simulink model "IP_Core_SS_Switch_and_PWM"  (R2021a)
settings: Solver=VariableStepAuto  StartTime=0.0  StopTime=0.001  RelTol=1e-3
values from neighbouring files (symbols this model uses):
  f_FPGA_clk = 100e6    (= 100000000)    [Init_IP_Core.m]
  T_FPGA_clk = 1/f_FPGA_clk    (= 1e-08)    [Init_IP_Core.m]
libraries: hdlsllib x4, simulink x2
(part 1 of 3)
settings Model: Creator=BHK  LastModifiedBy=micha
settings SolverCC: AlgebraicLoopSolver=TrustRegion
settings DataIOCC: ReturnWorkspaceOutputs=off
settings OptimizationCC: BlockReduction=off  ConditionallyExecuteInputs=off  DefaultParameterBehavior=Inlined
settings DebuggingCC: AlgebraicLoopMsg=error  SFMachineParentedDataDiag=warning  ArithmeticOperatorsInVariantConditions=warning
settings HardwareCC: ProdBitPerPointer=32  ProdBitPerSizeT=32  ProdBitPerPtrDiffT=32  ProdLargestAtomicFloat=None  ProdIntDivRoundTo=Undefined  ProdEndianess=Unspecified  ProdWordSize=32  ProdHWDeviceType=ASIC/FPGA->ASIC/FPGA  TargetBitPerPointer=64  TargetBitPerSizeT=64  TargetBitPerPtrDiffT=64  TargetLongLongMode=on  TargetIntDivRoundTo=Zero  TargetEndianess=LittleEndian  TargetWordSize=64  TargetHWDeviceType=Custom Processor->MATLAB Host Computer  ProdEqTarget=off
settings SFSimCC: SimUseLocalCustomCode=off  CustomCodeUndefinedFunction=UseInterfaceOnly
settings RTWCC: RTWUseLocalCustomCode=off

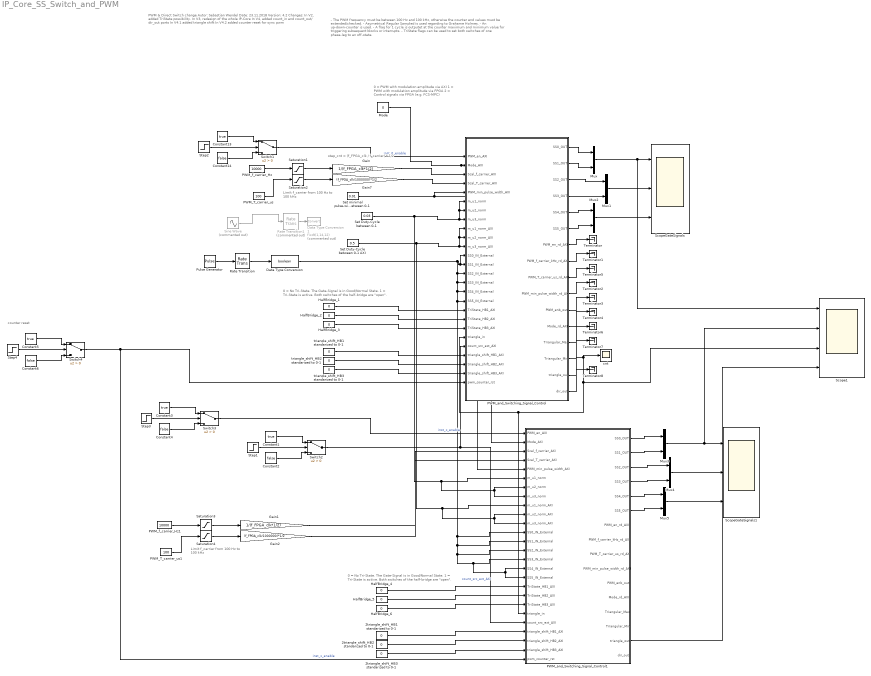
== system IP_Core_SS_Switch_and_PWM ==
  note: counter reset
  note: 0 = No Tri-State. The Gate-Signal is in Good/Normal State.
      | 1 = Tri-State is active. Both switches of the half-bridge are "open".
  note: PWM & Direct Switch change
      |
      | Autor: Sebastian Wendel
      | Date: 23.11.2018
      | Version: 4.2
      | Changes: In V2, added TriState possibility.
      | In V3, redesign of the whole IP-Core
      | In V4, added count_in and count_out/
      | dir_out ports
      | In V4.1 added triangle shift
      | In V4.2 added counter reset for sync pwm
  note: 0 = PWM with modulation amplitude via AXI
      | 1 = PWM with modulation amplitude via FPGA
      | 2 = Control signals via FPGA (e.g. FCS-MPC)
  note: step_cnt = (f_FPGA_clk / f_carrier) * 1/2
  note: Limit f_carrier from
      | 100 Hz to 100 kHz
  note: - The PWM frequency must be between 100 Hz and 100 kHz, otherwise the counter end values must be extended/checked.
      | - Asymetrical Regular Sampled is used regarding to Grahame Holmes.
      | - An up-down-counter is used.
      | - A flag for 1 cycle is outputet at the counter maximum and minimum value for triggering subsequent blocks or interrupts.
      | - TriState flags can be used to set both switches of one phase-leg to an off-state.
  note: 0 = No Tri-State. The Gate-Signal is in Good/Normal State.
      | 1 = Tri-State is active. Both switches of the half-bridge are "open".
  note: Limit f_carrier from
      | 100 Hz to 100 kHz
  2triangle_shift_HB1 standarized to 0-1 : Constant  Value=0  OutDataTypeStr=fixdt(0,18,17)  SampleTime=T_FPGA_clk
  2triangle_shift_HB2 standarized to 0-1 : Constant  Value=0  OutDataTypeStr=fixdt(0,18,17)  SampleTime=T_FPGA_clk
  2triangle_shift_HB3 standarized to 0-1 : Constant  Value=0  OutDataTypeStr=fixdt(0,18,17)  SampleTime=T_FPGA_clk
  Constant{1,3,5,13} (4 alike) : Constant  Value=true  SampleTime=T_FPGA_clk
  Constant{2,4,6,14} (4 alike) : Constant  Value=false  SampleTime=T_FPGA_clk
  Data Type Conversion : DataTypeConversion  OutDataTypeStr=boolean
  Data Type Conversion1 : DataTypeConversion  Commented=on  OutDataTypeStr=fixdt(1,14,12)
  Gain : Gain  Gain=1/(f_FPGA_clk*1/2)  OutDataTypeStr=fixdt(0,25,26)
  Gain1 : Gain  Gain=1/(f_FPGA_clk*1/2)  OutDataTypeStr=fixdt(0,25,26)
  Gain2 : Gain  Gain=(f_FPGA_clk/1000000)*1/2  OutDataTypeStr=fixdt(0,25,0)
  Gain7 : Gain  Gain=(f_FPGA_clk/1000000)*1/2  OutDataTypeStr=fixdt(0,25,0)
  HalfBridge_{1..6} (6 alike) : Constant  Value=0  OutDataTypeStr=fixdt(0,2,0)  SampleTime=T_FPGA_clk
  Mode : Constant  Value=0  OutDataTypeStr=fixdt(0,2,0)  SampleTime=T_FPGA_clk
  Mux{,1..5} (6 alike) : Mux  Inputs=2
  PWM_T_carrier_us : Constant  Value=100  OutDataTypeStr=uint32  SampleTime=T_FPGA_clk
  PWM_T_carrier_us1 : Constant  Value=100  OutDataTypeStr=uint32  SampleTime=T_FPGA_clk
  PWM_and_Switching_Signal_Control : Subsystem  TreatAsAtomicUnit=on
  PWM_and_Switching_Signal_Control1 : Subsystem  TreatAsAtomicUnit=on
  PWM_f_carrier_Hz : Constant  Value=10000  OutDataTypeStr=uint32  SampleTime=T_FPGA_clk
  PWM_f_carrier_Hz1 : Constant  Value=10000  OutDataTypeStr=uint32  SampleTime=T_FPGA_clk
  Pulse Generator : DiscretePulseGenerator  PulseType=Time based  Period=0.01  PulseWidth=5
  Rate Transition : RateTransition  OutPortSampleTime=T_FPGA_clk
  Rate Transition1 : RateTransition  Commented=on  OutPortSampleTime=T_FPGA_clk
  Saturation1 : Saturate  UpperLimit=100000  LowerLimit=100
  Saturation2 : Saturate  UpperLimit=10000  LowerLimit=10
  Saturation3 : Saturate  UpperLimit=100000  LowerLimit=100
  Saturation4 : Saturate  UpperLimit=10000  LowerLimit=10
  Scope1 : Scope  NumInputPorts=4
  ScopeGateSignals : Scope  NumInputPorts=3
  ScopeGateSignals1 : Scope  NumInputPorts=3
  Set Duty-Cycle between 0-1 : Constant  Value=0.03  OutDataTypeStr=fixdt(1,14,12)  SampleTime=T_FPGA_clk
  Set Duty-Cycle between 0-1 AXI : Constant  Value=0.5  OutDataTypeStr=fixdt(1,14,12)  SampleTime=T_FPGA_clk
  Set minimal pulse-width between 0-1 : Constant  Value=0.01  OutDataTypeStr=fixdt(1,18,16)  SampleTime=T_FPGA_clk
  Sine Wave : Sin  Commented=on  Frequency=500  SampleTime=0
  Step1 : Step  Time=0.002  After=0  SampleTime=T_FPGA_clk
  Step2 : Step  Time=0.00010  SampleTime=T_FPGA_clk
  Step3 : Step  Time=0.00019  SampleTime=T_FPGA_clk
  Step4 : Step  Time=0.0004  SampleTime=T_FPGA_clk
  Switch{1..4} (4 alike) : Switch  Criteria=u2 > Threshold
  Terminator{,1..8} (9 alike) : Terminator
  cnt : Scope
  triangle_shift_HB1 standarized to 0-1 : Constant  Value=0  OutDataTypeStr=fixdt(0,18,17)  SampleTime=T_FPGA_clk
  triangle_shift_HB2 standarized to 0-1 : Constant  Value=0  OutDataTypeStr=fixdt(0,18,17)  SampleTime=T_FPGA_clk
  triangle_shift_HB3 standarized to 0-1 : Constant  Value=0  OutDataTypeStr=fixdt(0,18,17)  SampleTime=T_FPGA_clk
  wires:
  Step2/1 -> Switch1/2
  Constant13/1 -> Switch1/1
  Constant14/1 -> Switch1/3
  Switch1/1 -> PWM_and_Switching_Signal_Control/1(PWM_en_AXI)  "inst_0_enable"
  Mode/1 -> PWM_and_Switching_Signal_Control1/2(Mode_AXI), PWM_and_Switching_Signal_Control/2(Mode_AXI)
  PWM_f_carrier_Hz/1 -> Saturation1/1
  Set minimal pulse-width between 0-1/1 -> PWM_and_Switching_Signal_Control1/5(PWM_min_pulse_width_AXI), PWM_and_Switching_Signal_Control/5(PWM_min_pulse_width_AXI)
  Sine Wave/1 -> Rate Transition1/1
  PWM_and_Switching_Signal_Control/7(PWM_en_rd_AXI) -> Terminator/1
  PWM_and_Switching_Signal_Control/8(PWM_f_carrier_kHz_rd_AXI) -> Terminator1/1
  PWM_and_Switching_Signal_Control/10(PWM_min_pulse_width_rd_AXI) -> Terminator2/1
  PWM_and_Switching_Signal_Control/11(PWM_enb_out) -> Terminator3/1
  PWM_and_Switching_Signal_Control/12(Mode_rd_AXI) -> Terminator4/1
  Set Duty-Cycle between 0-1 AXI/1 -> PWM_and_Switching_Signal_Control1/11(m_u3_norm_AXI), PWM_and_Switching_Signal_Control1/10(m_u2_norm_AXI), PWM_and_Switching_Signal_Control1/9(m_u1_norm_AXI), PWM_and_Switching_Signal_Control/9(m_u1_norm_AXI), PWM_and_Switching_Signal_Control/10(m_u2_norm_AXI), PWM_and_Switching_Signal_Control/11(m_u3_norm_AXI)
  PWM_and_Switching_Signal_Control/1(SS0_OUT) -> Mux/1
  PWM_and_Switching_Signal_Control/2(SS1_OUT) -> Mux/2
  Mux/1 -> Scope1/1, ScopeGateSignals/1
  PWM_and_Switching_Signal_Control/3(SS2_OUT) -> Mux1/1
  PWM_and_Switching_Signal_Control/4(SS3_OUT) -> Mux1/2
  PWM_and_Switching_Signal_Control/5(SS4_OUT) -> Mux2/1
  PWM_and_Switching_Signal_Control/6(SS5_OUT) -> Mux2/2
  Mux2/1 -> ScopeGateSignals/3
  Mux1/1 -> ScopeGateSignals/2
  PWM_T_carrier_us/1 -> Saturation2/1
  Rate Transition/1 -> Data Type Conversion/1
  Pulse Generator/1 -> Rate Transition/1
  PWM_and_Switching_Signal_Control/9(PWM_T_carrier_us_rd_AXI) -> Terminator5/1
  PWM_and_Switching_Signal_Control/13(Triangular_Max) -> Terminator6/1
  HalfBridge_3/1 -> PWM_and_Switching_Signal_Control/20(TriState_HB3_AXI)
  HalfBridge_2/1 -> PWM_and_Switching_Signal_Control/19(TriState_HB2_AXI)
  HalfBridge_1/1 -> PWM_and_Switching_Signal_Control/18(TriState_HB1_AXI)
  PWM_and_Switching_Signal_Control/14(Triangular_Min) -> Terminator7/1
  Gain/1 -> PWM_and_Switching_Signal_Control/3(Scal_f_carrier_AXI)
  Gain7/1 -> PWM_and_Switching_Signal_Control/4(Scal_T_carrier_AXI)
  Saturation1/1 -> Gain/1
  Saturation2/1 -> Gain7/1
  Rate Transition1/1 -> Data Type Conversion1/1
  Set Duty-Cycle between 0-1/1 -> PWM_and_Switching_Signal_Control/6(m_u1_norm), PWM_and_Switching_Signal_Control/7(m_u2_norm), PWM_and_Switching_Signal_Control/8(m_u3_norm), PWM_and_Switching_Signal_Control1/6(m_u1_norm), PWM_and_Switching_Signal_Control1/8(m_u3_norm), PWM_and_Switching_Signal_Control1/7(m_u2_norm)
  PWM_and_Switching_Signal_Control/16(dir_out) -> Terminator8/1
  Constant2/1 -> Switch2/3
  Step1/1 -> Switch2/2
  Constant1/1 -> Switch2/1
  Switch2/1 -> PWM_and_Switching_Signal_Control1/22(count_src_ext_AXI), PWM_and_Switching_Signal_Control/22(count_src_ext_AXI)  "count_src_ext_AXI"
  PWM_and_Switching_Signal_Control/15(triangle_out) -> cnt/1, PWM_and_Switching_Signal_Control/21(triangle_in), PWM_and_Switching_Signal_Control1/21(triangle_in), Scope1/3
  Data Type Conversion/1 -> PWM_and_Switching_Signal_Control/12(SS0_IN_External), PWM_and_Switching_Signal_Control/13(SS1_IN_External), PWM_and_Switching_Signal_Control1/12(SS0_IN_External), PWM_and_Switching_Signal_Control1/13(SS1_IN_External), PWM_and_Switching_Signal_Control1/14(SS2_IN_External), PWM_and_Switching_Signal_Control1/17(SS5_IN_External), PWM_and_Switching_Signal_Control1/16(SS4_IN_External), PWM_and_Switching_Signal_Control1/15(SS3_IN_External), PWM_and_Switching_Signal_Control/17(SS5_IN_External), PWM_and_Switching_Signal_Control/16(SS4_IN_External), PWM_and_Switching_Signal_Control/15(SS3_IN_External), PWM_and_Switching_Signal_Control/14(SS2_IN_External)
  HalfBridge_4/1 -> PWM_and_Switching_Signal_Control1/18(TriState_HB1_AXI)
  HalfBridge_6/1 -> PWM_and_Switching_Signal_Control1/20(TriState_HB3_AXI)
  HalfBridge_5/1 -> PWM_and_Switching_Signal_Control1/19(TriState_HB2_AXI)
  Mux3/1 -> ScopeGateSignals1/1, Scope1/2
  Mux5/1 -> ScopeGateSignals1/3
  Mux4/1 -> ScopeGateSignals1/2
  triangle_shift_HB1 standarized to 0-1/1 -> PWM_and_Switching_Signal_Control/23(triangle_shift_HB1_AXI)
  triangle_shift_HB2 standarized to 0-1/1 -> PWM_and_Switching_Signal_Control/24(triangle_shift_HB2_AXI)
  triangle_shift_HB3 standarized to 0-1/1 -> PWM_and_Switching_Signal_Control/25(triangle_shift_HB3_AXI)
  2triangle_shift_HB1 standarized to 0-1/1 -> PWM_and_Switching_Signal_Control1/23(triangle_shift_HB1_AXI)
  2triangle_shift_HB2 standarized to 0-1/1 -> PWM_and_Switching_Signal_Control1/24(triangle_shift_HB2_AXI)
  2triangle_shift_HB3 standarized to 0-1/1 -> PWM_and_Switching_Signal_Control1/25(triangle_shift_HB3_AXI)
  PWM_and_Switching_Signal_Control1/1(SS0_OUT) -> Mux3/1
  PWM_and_Switching_Signal_Control1/2(SS1_OUT) -> Mux3/2
  PWM_and_Switching_Signal_Control1/3(SS2_OUT) -> Mux4/1
  PWM_and_Switching_Signal_Control1/4(SS3_OUT) -> Mux4/2
  PWM_and_Switching_Signal_Control1/5(SS4_OUT) -> Mux5/1
  PWM_and_Switching_Signal_Control1/6(SS5_OUT) -> Mux5/2
  Step3/1 -> Switch3/2
  Constant4/1 -> Switch3/3
  Constant3/1 -> Switch3/1
  Switch3/1 -> PWM_and_Switching_Signal_Control1/1(PWM_en_AXI)  "inst_x_enable"
  Saturation3/1 -> Gain1/1
  PWM_f_carrier_Hz1/1 -> Saturation3/1
  Saturation4/1 -> Gain2/1
  PWM_T_carrier_us1/1 -> Saturation4/1
  Gain1/1 -> PWM_and_Switching_Signal_Control1/3(Scal_f_carrier_AXI)
  Gain2/1 -> PWM_and_Switching_Signal_Control1/4(Scal_T_carrier_AXI)
  PWM_and_Switching_Signal_Control1/15(triangle_out) -> Scope1/4
  Step4/1 -> Switch4/2
  Constant6/1 -> Switch4/3
  Constant5/1 -> Switch4/1
  Switch4/1 -> PWM_and_Switching_Signal_Control1/26(pwm_counter_rst), PWM_and_Switching_Signal_Control/26(pwm_counter_rst)  "inst_x_enable"

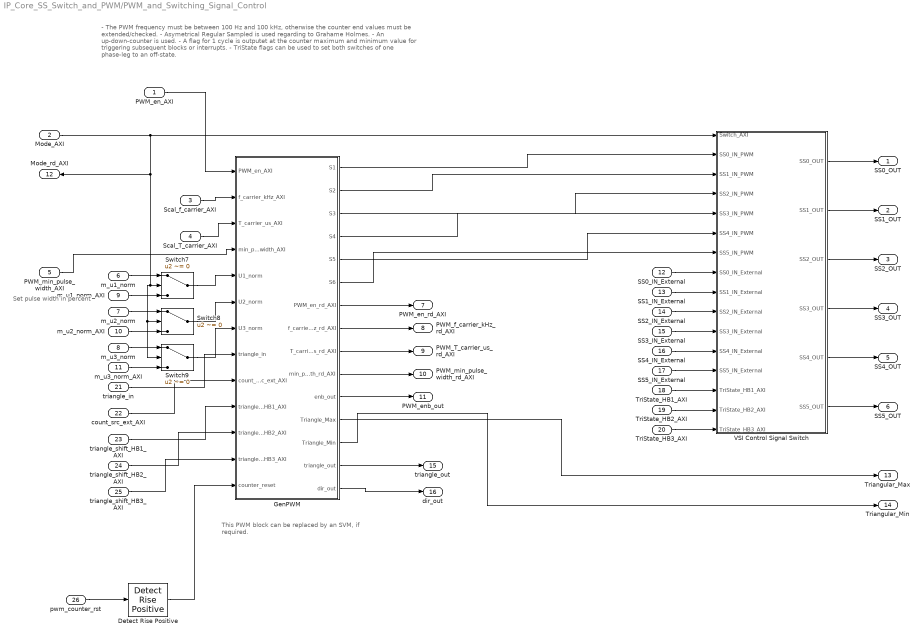
== system IP_Core_SS_Switch_and_PWM/PWM_and_Switching_Signal_Control ==
  note: This PWM block can be replaced by an SVM,
      | if required.
  note: - The PWM frequency must be between 100 Hz and 100 kHz, otherwise the counter end values must be extended/checked.
      | - Asymetrical Regular Sampled is used regarding to Grahame Holmes.
      | - An up-down-counter is used.
      | - A flag for 1 cycle is outputet at the counter maximum and minimum value for triggering subsequent blocks or interrupts.
      | - TriState flags can be used to set both switches of one phase-leg to an off-state.
  note: Set pulse width in percent
  PWM_en_AXI : Inport
  Mode_AXI : Inport  Port=2
  Scal_f_carrier_AXI : Inport  Port=3
  Scal_T_carrier_AXI : Inport  Port=4
  PWM_min_pulse_width_AXI : Inport  Port=5
  m_u1_norm : Inport  Port=6
  m_u2_norm : Inport  Port=7
  m_u3_norm : Inport  Port=8
  m_u1_norm_AXI : Inport  Port=9
  m_u2_norm_AXI : Inport  Port=10
  m_u3_norm_AXI : Inport  Port=11
  SS0_IN_External : Inport  Port=12
  SS1_IN_External : Inport  Port=13
  SS2_IN_External : Inport  Port=14
  SS3_IN_External : Inport  Port=15
  SS4_IN_External : Inport  Port=16
  SS5_IN_External : Inport  Port=17
  TriState_HB1_AXI : Inport  Port=18
  TriState_HB2_AXI : Inport  Port=19
  TriState_HB3_AXI : Inport  Port=20
  triangle_in : Inport  Port=21
  count_src_ext_AXI : Inport  Port=22
  triangle_shift_HB1_AXI : Inport  Port=23
  triangle_shift_HB2_AXI : Inport  Port=24
  triangle_shift_HB3_AXI : Inport  Port=25
  pwm_counter_rst : Inport  Port=26
  Detect Rise Positive : simulink/Logic and Bit Operations/Detect Rise Positive  vinit=0  OutDataTypeStr=boolean
  GenPWM : Subsystem  TreatAsAtomicUnit=on
  Switch7 : Switch  Criteria=u2 ~= 0
  Switch8 : Switch  Criteria=u2 ~= 0
  Switch9 : Switch  Criteria=u2 ~= 0
  VSI Control Signal Switch : Subsystem
  SS0_OUT : Outport  VectorParamsAs1DForOutWhenUnconnected=off
  SS1_OUT : Outport  Port=2  VectorParamsAs1DForOutWhenUnconnected=off
  SS2_OUT : Outport  Port=3  VectorParamsAs1DForOutWhenUnconnected=off
  SS3_OUT : Outport  Port=4  VectorParamsAs1DForOutWhenUnconnected=off
  SS4_OUT : Outport  Port=5  VectorParamsAs1DForOutWhenUnconnected=off
  SS5_OUT : Outport  Port=6  VectorParamsAs1DForOutWhenUnconnected=off
  PWM_en_rd_AXI : Outport  Port=7  VectorParamsAs1DForOutWhenUnconnected=off
  PWM_f_carrier_kHz_rd_AXI : Outport  Port=8  VectorParamsAs1DForOutWhenUnconnected=off
  PWM_T_carrier_us_rd_AXI : Outport  Port=9  VectorParamsAs1DForOutWhenUnconnected=off
  PWM_min_pulse_width_rd_AXI : Outport  Port=10  VectorParamsAs1DForOutWhenUnconnected=off
  PWM_enb_out : Outport  Port=11  VectorParamsAs1DForOutWhenUnconnected=off
  Mode_rd_AXI : Outport  Port=12  VectorParamsAs1DForOutWhenUnconnected=off
  Triangular_Max : Outport  Port=13  VectorParamsAs1DForOutWhenUnconnected=off
  Triangular_Min : Outport  Port=14  VectorParamsAs1DForOutWhenUnconnected=off
  triangle_out : Outport  Port=15  VectorParamsAs1DForOutWhenUnconnected=off
  dir_out : Outport  Port=16  VectorParamsAs1DForOutWhenUnconnected=off
  wires:
  VSI Control Signal Switch/1(SS0_OUT) -> SS0_OUT/1
  Mode_AXI/1 -> Mode_rd_AXI/1, Switch9/2, Switch8/2, Switch7/2, VSI Control Signal Switch/1(Switch_AXI)
  GenPWM/4(S4) -> VSI Control Signal Switch/5(SS3_IN_PWM)
  Scal_f_carrier_AXI/1 -> GenPWM/2(f_carrier_kHz_AXI)
  GenPWM/2(S2) -> VSI Control Signal Switch/3(SS1_IN_PWM)
  SS1_IN_External/1 -> VSI Control Signal Switch/9(SS1_IN_External)
  GenPWM/3(S3) -> VSI Control Signal Switch/4(SS2_IN_PWM)
  GenPWM/5(S5) -> VSI Control Signal Switch/6(SS4_IN_PWM)
  GenPWM/6(S6) -> VSI Control Signal Switch/7(SS5_IN_PWM)
  VSI Control Signal Switch/6(SS5_OUT) -> SS5_OUT/1
  GenPWM/1(S1) -> VSI Control Signal Switch/2(SS0_IN_PWM)
  GenPWM/11(enb_out) -> PWM_enb_out/1
  VSI Control Signal Switch/3(SS2_OUT) -> SS2_OUT/1
  SS3_IN_External/1 -> VSI Control Signal Switch/11(SS3_IN_External)
  SS0_IN_External/1 -> VSI Control Signal Switch/8(SS0_IN_External)
  VSI Control Signal Switch/2(SS1_OUT) -> SS1_OUT/1
  SS4_IN_External/1 -> VSI Control Signal Switch/12(SS4_IN_External)
  SS5_IN_External/1 -> VSI Control Signal Switch/13(SS5_IN_External)
  VSI Control Signal Switch/5(SS4_OUT) -> SS4_OUT/1
  PWM_min_pulse_width_AXI/1 -> GenPWM/4(min_pulse_width_AXI)
  SS2_IN_External/1 -> VSI Control Signal Switch/10(SS2_IN_External)
  VSI Control Signal Switch/4(SS3_OUT) -> SS3_OUT/1
  Switch9/1 -> GenPWM/7(U3_norm)
  m_u1_norm_AXI/1 -> Switch7/3
  m_u1_norm/1 -> Switch7/1
  m_u2_norm/1 -> Switch8/1
  m_u2_norm_AXI/1 -> Switch8/3
  m_u3_norm/1 -> Switch9/1
  m_u3_norm_AXI/1 -> Switch9/3
  GenPWM/7(PWM_en_rd_AXI) -> PWM_en_rd_AXI/1
  GenPWM/8(f_carrier_kHz_rd_AXI) -> PWM_f_carrier_kHz_rd_AXI/1
  GenPWM/10(min_pulse_width_rd_AXI) -> PWM_min_pulse_width_rd_AXI/1
  GenPWM/9(T_carrier_us_rd_AXI) -> PWM_T_carrier_us_rd_AXI/1
  Switch8/1 -> GenPWM/6(U2_norm)
  Switch7/1 -> GenPWM/5(U1_norm)
  Scal_T_carrier_AXI/1 -> GenPWM/3(T_carrier_us_AXI)
  GenPWM/12(Triangle_Max) -> Triangular_Max/1
  TriState_HB1_AXI/1 -> VSI Control Signal Switch/14(TriState_HB1_AXI)
  TriState_HB2_AXI/1 -> VSI Control Signal Switch/15(TriState_HB2_AXI)
  TriState_HB3_AXI/1 -> VSI Control Signal Switch/16(TriState_HB3_AXI)
  GenPWM/13(Triangle_Min) -> Triangular_Min/1
  triangle_in/1 -> GenPWM/8(triangle_in)
  GenPWM/14(triangle_out) -> triangle_out/1
  GenPWM/15(dir_out) -> dir_out/1
  count_src_ext_AXI/1 -> GenPWM/9(count_src_ext_AXI)
  triangle_shift_HB1_AXI/1 -> GenPWM/10(triangle_shift_HB1_AXI)
  triangle_shift_HB3_AXI/1 -> GenPWM/12(triangle_shift_HB3_AXI)
  triangle_shift_HB2_AXI/1 -> GenPWM/11(triangle_shift_HB2_AXI)
  PWM_en_AXI/1 -> GenPWM/1(PWM_en_AXI)
  pwm_counter_rst/1 -> Detect Rise Positive/1
  Detect Rise Positive/1 -> GenPWM/13(counter_reset)

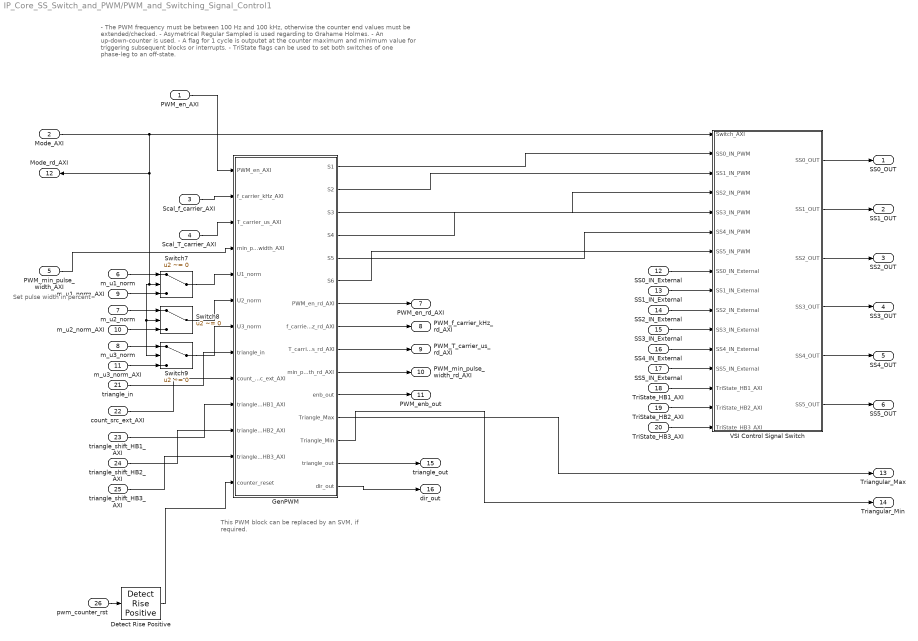
== system IP_Core_SS_Switch_and_PWM/PWM_and_Switching_Signal_Control1 ==
  note: This PWM block can be replaced by an SVM,
      | if required.
  note: - The PWM frequency must be between 100 Hz and 100 kHz, otherwise the counter end values must be extended/checked.
      | - Asymetrical Regular Sampled is used regarding to Grahame Holmes.
      | - An up-down-counter is used.
      | - A flag for 1 cycle is outputet at the counter maximum and minimum value for triggering subsequent blocks or interrupts.
      | - TriState flags can be used to set both switches of one phase-leg to an off-state.
  note: Set pulse width in percent
  PWM_en_AXI : Inport
  Mode_AXI : Inport  Port=2
  Scal_f_carrier_AXI : Inport  Port=3
  Scal_T_carrier_AXI : Inport  Port=4
  PWM_min_pulse_width_AXI : Inport  Port=5
  m_u1_norm : Inport  Port=6
  m_u2_norm : Inport  Port=7
  m_u3_norm : Inport  Port=8
  m_u1_norm_AXI : Inport  Port=9
  m_u2_norm_AXI : Inport  Port=10
  m_u3_norm_AXI : Inport  Port=11
  SS0_IN_External : Inport  Port=12
  SS1_IN_External : Inport  Port=13
  SS2_IN_External : Inport  Port=14
  SS3_IN_External : Inport  Port=15
  SS4_IN_External : Inport  Port=16
  SS5_IN_External : Inport  Port=17
  TriState_HB1_AXI : Inport  Port=18
  TriState_HB2_AXI : Inport  Port=19
  TriState_HB3_AXI : Inport  Port=20
  triangle_in : Inport  Port=21
  count_src_ext_AXI : Inport  Port=22
  triangle_shift_HB1_AXI : Inport  Port=23
  triangle_shift_HB2_AXI : Inport  Port=24
  triangle_shift_HB3_AXI : Inport  Port=25
  pwm_counter_rst : Inport  Port=26
  Detect Rise Positive : simulink/Logic and Bit Operations/Detect Rise Positive  vinit=0  OutDataTypeStr=boolean
  GenPWM : Subsystem  TreatAsAtomicUnit=on
  Switch7 : Switch  Criteria=u2 ~= 0
  Switch8 : Switch  Criteria=u2 ~= 0
  Switch9 : Switch  Criteria=u2 ~= 0
  VSI Control Signal Switch : Subsystem
  SS0_OUT : Outport  VectorParamsAs1DForOutWhenUnconnected=off
  SS1_OUT : Outport  Port=2  VectorParamsAs1DForOutWhenUnconnected=off
  SS2_OUT : Outport  Port=3  VectorParamsAs1DForOutWhenUnconnected=off
  SS3_OUT : Outport  Port=4  VectorParamsAs1DForOutWhenUnconnected=off
  SS4_OUT : Outport  Port=5  VectorParamsAs1DForOutWhenUnconnected=off
  SS5_OUT : Outport  Port=6  VectorParamsAs1DForOutWhenUnconnected=off
  PWM_en_rd_AXI : Outport  Port=7  VectorParamsAs1DForOutWhenUnconnected=off
  PWM_f_carrier_kHz_rd_AXI : Outport  Port=8  VectorParamsAs1DForOutWhenUnconnected=off
  PWM_T_carrier_us_rd_AXI : Outport  Port=9  VectorParamsAs1DForOutWhenUnconnected=off
  PWM_min_pulse_width_rd_AXI : Outport  Port=10  VectorParamsAs1DForOutWhenUnconnected=off
  PWM_enb_out : Outport  Port=11  VectorParamsAs1DForOutWhenUnconnected=off
  Mode_rd_AXI : Outport  Port=12  VectorParamsAs1DForOutWhenUnconnected=off
  Triangular_Max : Outport  Port=13  VectorParamsAs1DForOutWhenUnconnected=off
  Triangular_Min : Outport  Port=14  VectorParamsAs1DForOutWhenUnconnected=off
  triangle_out : Outport  Port=15  VectorParamsAs1DForOutWhenUnconnected=off
  dir_out : Outport  Port=16  VectorParamsAs1DForOutWhenUnconnected=off
  wires:
  VSI Control Signal Switch/1(SS0_OUT) -> SS0_OUT/1
  Mode_AXI/1 -> Mode_rd_AXI/1, Switch9/2, Switch8/2, Switch7/2, VSI Control Signal Switch/1(Switch_AXI)
  GenPWM/4(S4) -> VSI Control Signal Switch/5(SS3_IN_PWM)
  Scal_f_carrier_AXI/1 -> GenPWM/2(f_carrier_kHz_AXI)
  GenPWM/2(S2) -> VSI Control Signal Switch/3(SS1_IN_PWM)
  SS1_IN_External/1 -> VSI Control Signal Switch/9(SS1_IN_External)
  GenPWM/3(S3) -> VSI Control Signal Switch/4(SS2_IN_PWM)
  GenPWM/5(S5) -> VSI Control Signal Switch/6(SS4_IN_PWM)
  GenPWM/6(S6) -> VSI Control Signal Switch/7(SS5_IN_PWM)
  VSI Control Signal Switch/6(SS5_OUT) -> SS5_OUT/1
  GenPWM/1(S1) -> VSI Control Signal Switch/2(SS0_IN_PWM)
  GenPWM/11(enb_out) -> PWM_enb_out/1
  VSI Control Signal Switch/3(SS2_OUT) -> SS2_OUT/1
  SS3_IN_External/1 -> VSI Control Signal Switch/11(SS3_IN_External)
  SS0_IN_External/1 -> VSI Control Signal Switch/8(SS0_IN_External)
  VSI Control Signal Switch/2(SS1_OUT) -> SS1_OUT/1
  SS4_IN_External/1 -> VSI Control Signal Switch/12(SS4_IN_External)
  SS5_IN_External/1 -> VSI Control Signal Switch/13(SS5_IN_External)
  VSI Control Signal Switch/5(SS4_OUT) -> SS4_OUT/1
  PWM_min_pulse_width_AXI/1 -> GenPWM/4(min_pulse_width_AXI)
  SS2_IN_External/1 -> VSI Control Signal Switch/10(SS2_IN_External)
  VSI Control Signal Switch/4(SS3_OUT) -> SS3_OUT/1
  Switch9/1 -> GenPWM/7(U3_norm)
  m_u1_norm_AXI/1 -> Switch7/3
  m_u1_norm/1 -> Switch7/1
  m_u2_norm/1 -> Switch8/1
  m_u2_norm_AXI/1 -> Switch8/3
  m_u3_norm/1 -> Switch9/1
  m_u3_norm_AXI/1 -> Switch9/3
  GenPWM/7(PWM_en_rd_AXI) -> PWM_en_rd_AXI/1
  GenPWM/8(f_carrier_kHz_rd_AXI) -> PWM_f_carrier_kHz_rd_AXI/1
  GenPWM/10(min_pulse_width_rd_AXI) -> PWM_min_pulse_width_rd_AXI/1
  GenPWM/9(T_carrier_us_rd_AXI) -> PWM_T_carrier_us_rd_AXI/1
  Switch8/1 -> GenPWM/6(U2_norm)
  Switch7/1 -> GenPWM/5(U1_norm)
  Scal_T_carrier_AXI/1 -> GenPWM/3(T_carrier_us_AXI)
  GenPWM/12(Triangle_Max) -> Triangular_Max/1
  TriState_HB1_AXI/1 -> VSI Control Signal Switch/14(TriState_HB1_AXI)
  TriState_HB2_AXI/1 -> VSI Control Signal Switch/15(TriState_HB2_AXI)
  TriState_HB3_AXI/1 -> VSI Control Signal Switch/16(TriState_HB3_AXI)
  GenPWM/13(Triangle_Min) -> Triangular_Min/1
  triangle_in/1 -> GenPWM/8(triangle_in)
  GenPWM/14(triangle_out) -> triangle_out/1
  GenPWM/15(dir_out) -> dir_out/1
  triangle_shift_HB1_AXI/1 -> GenPWM/10(triangle_shift_HB1_AXI)
  triangle_shift_HB3_AXI/1 -> GenPWM/12(triangle_shift_HB3_AXI)
  triangle_shift_HB2_AXI/1 -> GenPWM/11(triangle_shift_HB2_AXI)
  pwm_counter_rst/1 -> Detect Rise Positive/1
  PWM_en_AXI/1 -> GenPWM/1(PWM_en_AXI)
  count_src_ext_AXI/1 -> GenPWM/9(count_src_ext_AXI)
  Detect Rise Positive/1 -> GenPWM/13(counter_reset)

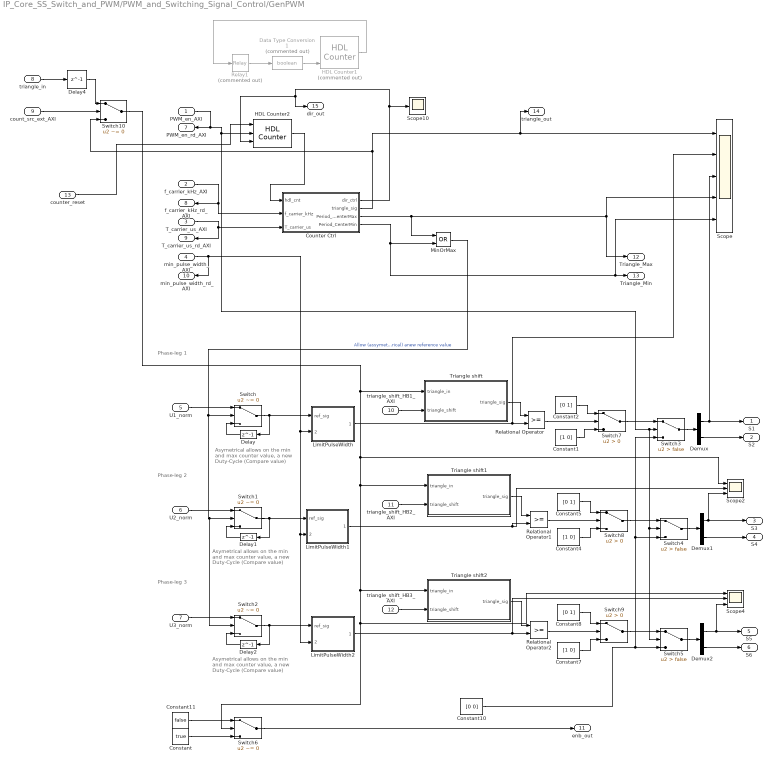
== system IP_Core_SS_Switch_and_PWM/PWM_and_Switching_Signal_Control/GenPWM ==
  note: Asymetrical allows on the min
      |  and max counter value, a new
      |  Duty-Cycle (Compare value)
  note: Phase-leg 1
  note: Phase-leg 2
  note: Phase-leg 3
  note: Asymetrical allows on the min
      |  and max counter value, a new
      |  Duty-Cycle (Compare value)
  note: Asymetrical allows on the min
      |  and max counter value, a new
      |  Duty-Cycle (Compare value)
  PWM_en_AXI : Inport
  f_carrier_kHz_AXI : Inport  Port=2
  T_carrier_us_AXI : Inport  Port=3
  min_pulse_width_AXI : Inport  Port=4
  U1_norm : Inport  Port=5
  U2_norm : Inport  Port=6
  U3_norm : Inport  Port=7
  triangle_in : Inport  Port=8
  count_src_ext_AXI : Inport  Port=9
  triangle_shift_HB1_AXI : Inport  Port=10
  triangle_shift_HB2_AXI : Inport  Port=11
  triangle_shift_HB3_AXI : Inport  Port=12
  counter_reset : Inport  Port=13
  Constant : Constant  Value=true  SampleTime=T_FPGA_clk
  Constant1 : Constant  Value=[1 0]  OutDataTypeStr=fixdt(0,1,0)  SampleTime=T_FPGA_clk
  Constant10 : Constant  Value=[0 0]  OutDataTypeStr=fixdt(0,1,0)  SampleTime=T_FPGA_clk
  Constant11 : Constant  Value=false  SampleTime=T_FPGA_clk
  Constant2 : Constant  Value=[0 1]  OutDataTypeStr=fixdt(0,1,0)  SampleTime=T_FPGA_clk
  Constant4 : Constant  Value=[1 0]  OutDataTypeStr=fixdt(0,1,0)  SampleTime=T_FPGA_clk
  Constant5 : Constant  Value=[0 1]  OutDataTypeStr=fixdt(0,1,0)  SampleTime=T_FPGA_clk
  Constant7 : Constant  Value=[1 0]  OutDataTypeStr=fixdt(0,1,0)  SampleTime=T_FPGA_clk
  Constant8 : Constant  Value=[0 1]  OutDataTypeStr=fixdt(0,1,0)  SampleTime=T_FPGA_clk
  Counter Ctrl : Subsystem
  Data Type Conversion1 : DataTypeConversion  Commented=on  OutDataTypeStr=boolean
  Delay{,1..2,4} (4 alike) : Delay  DelayLength=1
  Demux : Demux  Outputs=2
  Demux1 : Demux  Outputs=2
  Demux2 : Demux  Outputs=2
  HDL Counter1 : hdlsllib/Sources/HDL Counter  Commented=on  CountType=Free running  CountInit=0  CountStep=1  CountMax=100  CountFromType=Initial value  CountFrom=0  CountResetPort=on  CountLoadPort=off  CountEnbPort=on  CountDirPort=on  CountHitOutputPort=off  CountDataType=Signed  CountWordLen=8  CountFracLen=0  CountSampTime=Ts
  HDL Counter2 : hdlsllib/Sources/HDL Counter  CountType=Free running  CountInit=0  CountStep=1  CountMax=100  CountFromType=Initial value  CountFrom=0  CountResetPort=on  CountLoadPort=off  CountEnbPort=on  CountDirPort=on  CountHitOutputPort=off  CountDataType=Unsigned  CountWordLen=20  CountFracLen=0  CountSampTime=1
  LimitPulseWidth : Subsystem
  LimitPulseWidth1 : Subsystem
  LimitPulseWidth2 : Subsystem
  MinOrMax : Logic  Operator=OR  AllPortsSameDT=off  OutDataTypeStr=boolean
  Relational Operator : RelationalOperator  OutDataTypeStr=boolean  RndMeth=Nearest
  Relational Operator1 : RelationalOperator  OutDataTypeStr=boolean  RndMeth=Nearest
  Relational Operator2 : RelationalOperator  OutDataTypeStr=boolean  RndMeth=Nearest
  Relay1 : Relay  Commented=on  OnSwitchValue=100  OffSwitchValue=0  OnOutputValue=0  OffOutputValue=1
  Scope : Scope  NumInputPorts=5
  Scope10 : Scope
  Scope2 : Scope  NumInputPorts=3
  Scope4 : Scope  NumInputPorts=3
  Switch : Switch  Criteria=u2 ~= 0  Threshold=1
  Switch1 : Switch  Criteria=u2 ~= 0
  Switch10 : Switch  Criteria=u2 ~= 0  Threshold=1
  Switch2 : Switch  Criteria=u2 ~= 0
  Switch3 : Switch  Criteria=u2 > Threshold  Threshold=false
  Switch4 : Switch  Criteria=u2 > Threshold  Threshold=false
  Switch5 : Switch  Criteria=u2 > Threshold  Threshold=false
  Switch6 : Switch  Criteria=u2 ~= 0
  Switch7 : Switch  Criteria=u2 > Threshold
  Switch8 : Switch  Criteria=u2 > Threshold
  Switch9 : Switch  Criteria=u2 > Threshold
  Triangle shift : Subsystem
  Triangle shift1 : Subsystem
  Triangle shift2 : Subsystem
  S1 : Outport  VectorParamsAs1DForOutWhenUnconnected=off
  S2 : Outport  Port=2  VectorParamsAs1DForOutWhenUnconnected=off
  S3 : Outport  Port=3  VectorParamsAs1DForOutWhenUnconnected=off
  S4 : Outport  Port=4  VectorParamsAs1DForOutWhenUnconnected=off
  S5 : Outport  Port=5  VectorParamsAs1DForOutWhenUnconnected=off
  S6 : Outport  Port=6  VectorParamsAs1DForOutWhenUnconnected=off
  PWM_en_rd_AXI : Outport  Port=7  VectorParamsAs1DForOutWhenUnconnected=off
  f_carrier_kHz_rd_AXI : Outport  Port=8  VectorParamsAs1DForOutWhenUnconnected=off
  T_carrier_us_rd_AXI : Outport  Port=9  VectorParamsAs1DForOutWhenUnconnected=off
  min_pulse_width_rd_AXI : Outport  Port=10  VectorParamsAs1DForOutWhenUnconnected=off
  enb_out : Outport  Port=11  VectorParamsAs1DForOutWhenUnconnected=off
  Triangle_Max : Outport  Port=12  VectorParamsAs1DForOutWhenUnconnected=off
  Triangle_Min : Outport  Port=13  VectorParamsAs1DForOutWhenUnconnected=off
  triangle_out : Outport  Port=14  VectorParamsAs1DForOutWhenUnconnected=off
  dir_out : Outport  Port=15  VectorParamsAs1DForOutWhenUnconnected=off
  wires:
  Constant7/1 -> Switch9/3
  Demux2/2 -> S6/1
  Constant8/1 -> Switch9/1
  Relational Operator2/1 -> Switch9/2
  Switch9/1 -> Switch5/1
  Demux/2 -> S2/1
  Relational Operator/1 -> Switch7/2
  Demux1/2 -> S4/1
  Constant5/1 -> Switch8/1
  Relational Operator1/1 -> Switch8/2
  Constant4/1 -> Switch8/3
  Constant1/1 -> Switch7/3
  Constant2/1 -> Switch7/1
  LimitPulseWidth/1(ref_sig_limit) -> Scope/2, Relational Operator/2
  LimitPulseWidth1/1(ref_sig_limit) -> Scope2/2, Relational Operator1/2
  LimitPulseWidth2/1(ref_sig_limit) -> Scope4/2, Relational Operator2/2
  Counter Ctrl/2(triangle_sig) -> triangle_out/1, Scope/1, Switch10/3
  PWM_en_AXI/1 -> Switch3/2, Switch4/2, Switch5/2, HDL Counter2/2, PWM_en_rd_AXI/1
  Delay/1 -> Switch/3
  Delay1/1 -> Switch1/3
  Delay2/1 -> Switch2/3
  Switch5/1 -> Demux2/1
  Switch8/1 -> Switch4/1
  Switch4/1 -> Demux1/1
  Switch3/1 -> Demux/1
  Constant10/1 -> Switch5/3, Switch3/3, Switch4/3
  U1_norm/1 -> Switch/1
  U3_norm/1 -> Switch2/1
  U2_norm/1 -> Switch1/1
  Counter Ctrl/1(dir_ctrl) -> dir_out/1, HDL Counter2/3, Scope10/1
  f_carrier_kHz_AXI/1 -> f_carrier_kHz_rd_AXI/1, Counter Ctrl/2(f_carrier_kHz)
  Relay1/1 -> Data Type Conversion1/1
  Data Type Conversion1/1 -> HDL Counter1/3
  HDL Counter1/1 -> Relay1/1
  Switch/1 -> Delay/1, LimitPulseWidth/1(ref_sig)
  Switch1/1 -> LimitPulseWidth1/1(ref_sig), Delay1/1
  Switch2/1 -> LimitPulseWidth2/1(ref_sig), Delay2/1
  Demux/1 -> Scope/3, S1/1
  Switch6/1 -> enb_out/1
  Constant11/1 -> Switch6/1
  Constant/1 -> Switch6/3
  Demux1/1 -> Scope2/3, S3/1
  Demux2/1 -> Scope4/3, S5/1
  T_carrier_us_AXI/1 -> T_carrier_us_rd_AXI/1, Counter Ctrl/3(T_carrier_us)
  Switch7/1 -> Switch3/1
  min_pulse_width_AXI/1 -> LimitPulseWidth/2(min_pulse_width), LimitPulseWidth2/2(min_pulse_width), LimitPulseWidth1/2(min_pulse_width), min_pulse_width_rd_AXI/1
  Counter Ctrl/3(Period_CenterMax) -> MinOrMax/1, Triangle_Max/1, Scope/4
  Counter Ctrl/4(Period_CenterMin) -> MinOrMax/2, Scope/5, Triangle_Min/1
  MinOrMax/1 -> Switch1/2, Switch2/2, Switch/2  "Allow (assymetrical) anew reference value"
  triangle_in/1 -> Delay4/1
  count_src_ext_AXI/1 -> Switch10/2
  HDL Counter2/1 -> Counter Ctrl/1(hdl_cnt)
  Delay4/1 -> Switch10/1
  triangle_shift_HB1_AXI/1 -> Triangle shift/2(triangle_shift)
  Triangle shift/1(triangle_sig) -> Relational Operator/1
  Triangle shift1/1(triangle_sig) -> Relational Operator1/1
  Switch10/1 -> Triangle shift/1(triangle_in), Triangle shift1/1(triangle_in), Triangle shift2/1(triangle_in), Scope4/1, Switch6/2, Scope2/1
  triangle_shift_HB2_AXI/1 -> Triangle shift1/2(triangle_shift)
  Triangle shift2/1(triangle_sig) -> Relational Operator2/1
  triangle_shift_HB3_AXI/1 -> Triangle shift2/2(triangle_shift)
  counter_reset/1 -> HDL Counter2/1

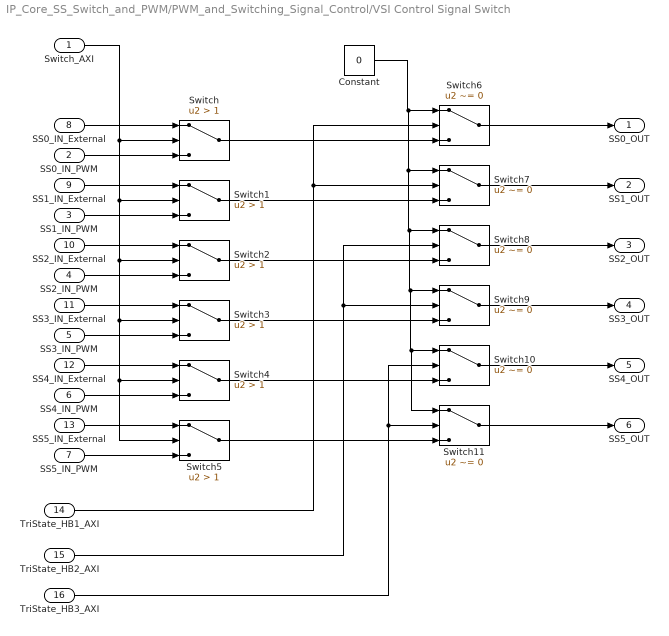
== system IP_Core_SS_Switch_and_PWM/PWM_and_Switching_Signal_Control/VSI Control Signal Switch ==
  Switch_AXI : Inport
  SS0_IN_PWM : Inport  Port=2
  SS1_IN_PWM : Inport  Port=3
  SS2_IN_PWM : Inport  Port=4
  SS3_IN_PWM : Inport  Port=5
  SS4_IN_PWM : Inport  Port=6
  SS5_IN_PWM : Inport  Port=7
  SS0_IN_External : Inport  Port=8
  SS1_IN_External : Inport  Port=9
  SS2_IN_External : Inport  Port=10
  SS3_IN_External : Inport  Port=11
  SS4_IN_External : Inport  Port=12
  SS5_IN_External : Inport  Port=13
  TriState_HB1_AXI : Inport  Port=14
  TriState_HB2_AXI : Inport  Port=15
  TriState_HB3_AXI : Inport  Port=16
  Constant : Constant  Value=0  OutDataTypeStr=boolean  SampleTime=T_FPGA_clk
  Switch{,1..5} (6 alike) : Switch  Criteria=u2 > Threshold  Threshold=1
  Switch{6..11} (6 alike) : Switch  Criteria=u2 ~= 0  Threshold=1
  SS0_OUT : Outport  VectorParamsAs1DForOutWhenUnconnected=off
  SS1_OUT : Outport  Port=2  VectorParamsAs1DForOutWhenUnconnected=off
  SS2_OUT : Outport  Port=3  VectorParamsAs1DForOutWhenUnconnected=off
  SS3_OUT : Outport  Port=4  VectorParamsAs1DForOutWhenUnconnected=off
  SS4_OUT : Outport  Port=5  VectorParamsAs1DForOutWhenUnconnected=off
  SS5_OUT : Outport  Port=6  VectorParamsAs1DForOutWhenUnconnected=off
  wires:
  Switch_AXI/1 -> Switch4/2, Switch5/2, Switch3/2, Switch2/2, Switch1/2, Switch/2
  Switch5/1 -> Switch11/3
  Switch/1 -> Switch6/3
  Switch3/1 -> Switch9/3
  Switch2/1 -> Switch8/3
  Switch1/1 -> Switch7/3
  Switch4/1 -> Switch10/3
  SS0_IN_PWM/1 -> Switch/3
  SS0_IN_External/1 -> Switch/1
  SS1_IN_External/1 -> Switch1/1
  SS1_IN_PWM/1 -> Switch1/3
  SS2_IN_External/1 -> Switch2/1
  SS2_IN_PWM/1 -> Switch2/3
  SS3_IN_External/1 -> Switch3/1
  SS3_IN_PWM/1 -> Switch3/3
  SS4_IN_External/1 -> Switch4/1
  SS4_IN_PWM/1 -> Switch4/3
  SS5_IN_External/1 -> Switch5/1
  SS5_IN_PWM/1 -> Switch5/3
  TriState_HB3_AXI/1 -> Switch10/2, Switch11/2
  TriState_HB2_AXI/1 -> Switch8/2, Switch9/2
  TriState_HB1_AXI/1 -> Switch6/2, Switch7/2
  Switch11/1 -> SS5_OUT/1
  Switch10/1 -> SS4_OUT/1
  Switch9/1 -> SS3_OUT/1
  Switch8/1 -> SS2_OUT/1
  Switch7/1 -> SS1_OUT/1
  Switch6/1 -> SS0_OUT/1
  Constant/1 -> Switch11/1, Switch10/1, Switch9/1, Switch8/1, Switch7/1, Switch6/1

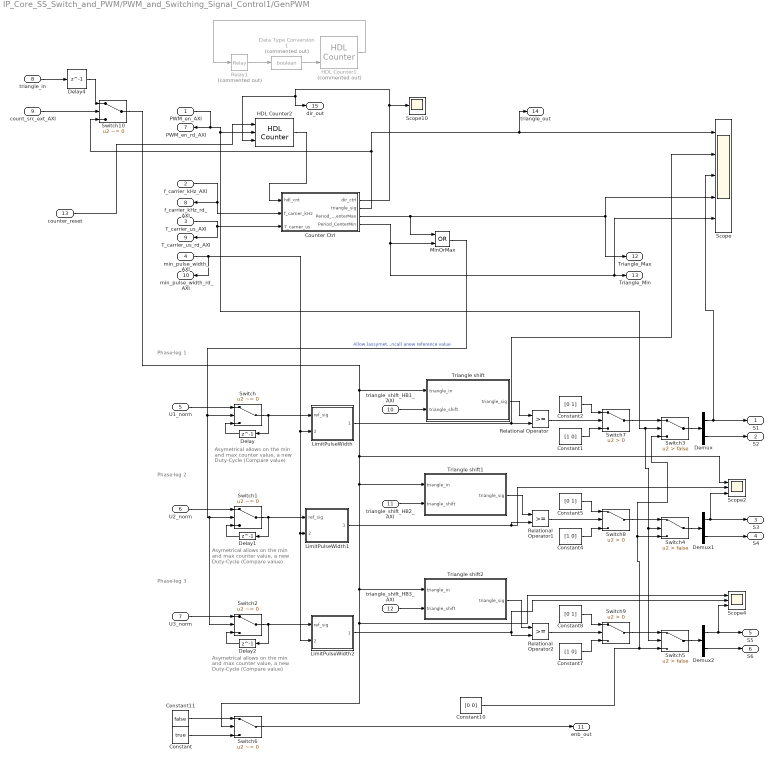
== system IP_Core_SS_Switch_and_PWM/PWM_and_Switching_Signal_Control1/GenPWM ==
  note: Asymetrical allows on the min
      |  and max counter value, a new
      |  Duty-Cycle (Compare value)
  note: Phase-leg 1
  note: Phase-leg 2
  note: Phase-leg 3
  note: Asymetrical allows on the min
      |  and max counter value, a new
      |  Duty-Cycle (Compare value)
  note: Asymetrical allows on the min
      |  and max counter value, a new
      |  Duty-Cycle (Compare value)
  PWM_en_AXI : Inport
  f_carrier_kHz_AXI : Inport  Port=2
  T_carrier_us_AXI : Inport  Port=3
  min_pulse_width_AXI : Inport  Port=4
  U1_norm : Inport  Port=5
  U2_norm : Inport  Port=6
  U3_norm : Inport  Port=7
  triangle_in : Inport  Port=8
  count_src_ext_AXI : Inport  Port=9
  triangle_shift_HB1_AXI : Inport  Port=10
  triangle_shift_HB2_AXI : Inport  Port=11
  triangle_shift_HB3_AXI : Inport  Port=12
  counter_reset : Inport  Port=13
  Constant : Constant  Value=true  SampleTime=T_FPGA_clk
  Constant1 : Constant  Value=[1 0]  OutDataTypeStr=fixdt(0,1,0)  SampleTime=T_FPGA_clk
  Constant10 : Constant  Value=[0 0]  OutDataTypeStr=fixdt(0,1,0)  SampleTime=T_FPGA_clk
  Constant11 : Constant  Value=false  SampleTime=T_FPGA_clk
  Constant2 : Constant  Value=[0 1]  OutDataTypeStr=fixdt(0,1,0)  SampleTime=T_FPGA_clk
  Constant4 : Constant  Value=[1 0]  OutDataTypeStr=fixdt(0,1,0)  SampleTime=T_FPGA_clk
  Constant5 : Constant  Value=[0 1]  OutDataTypeStr=fixdt(0,1,0)  SampleTime=T_FPGA_clk
  Constant7 : Constant  Value=[1 0]  OutDataTypeStr=fixdt(0,1,0)  SampleTime=T_FPGA_clk
  Constant8 : Constant  Value=[0 1]  OutDataTypeStr=fixdt(0,1,0)  SampleTime=T_FPGA_clk
  Counter Ctrl : Subsystem
  Data Type Conversion1 : DataTypeConversion  Commented=on  OutDataTypeStr=boolean
  Delay{,1..2,4} (4 alike) : Delay  DelayLength=1
  Demux : Demux  Outputs=2
  Demux1 : Demux  Outputs=2
  Demux2 : Demux  Outputs=2
  HDL Counter1 : hdlsllib/Sources/HDL Counter  Commented=on  CountType=Free running  CountInit=0  CountStep=1  CountMax=100  CountFromType=Initial value  CountFrom=0  CountResetPort=on  CountLoadPort=off  CountEnbPort=on  CountDirPort=on  CountHitOutputPort=off  CountDataType=Signed  CountWordLen=8  CountFracLen=0  CountSampTime=Ts
  HDL Counter2 : hdlsllib/Sources/HDL Counter  CountType=Free running  CountInit=0  CountStep=1  CountMax=100  CountFromType=Initial value  CountFrom=0  CountResetPort=on  CountLoadPort=off  CountEnbPort=on  CountDirPort=on  CountHitOutputPort=off  CountDataType=Unsigned  CountWordLen=20  CountFracLen=0  CountSampTime=1
  LimitPulseWidth : Subsystem
  LimitPulseWidth1 : Subsystem
  LimitPulseWidth2 : Subsystem
  MinOrMax : Logic  Operator=OR  AllPortsSameDT=off  OutDataTypeStr=boolean
  Relational Operator : RelationalOperator  OutDataTypeStr=boolean  RndMeth=Nearest
  Relational Operator1 : RelationalOperator  OutDataTypeStr=boolean  RndMeth=Nearest
  Relational Operator2 : RelationalOperator  OutDataTypeStr=boolean  RndMeth=Nearest
  Relay1 : Relay  Commented=on  OnSwitchValue=100  OffSwitchValue=0  OnOutputValue=0  OffOutputValue=1
  Scope : Scope  NumInputPorts=5
  Scope10 : Scope
  Scope2 : Scope  NumInputPorts=3
  Scope4 : Scope  NumInputPorts=3
  Switch : Switch  Criteria=u2 ~= 0  Threshold=1
  Switch1 : Switch  Criteria=u2 ~= 0
  Switch10 : Switch  Criteria=u2 ~= 0  Threshold=1
  Switch2 : Switch  Criteria=u2 ~= 0
  Switch3 : Switch  Criteria=u2 > Threshold  Threshold=false
  Switch4 : Switch  Criteria=u2 > Threshold  Threshold=false
  Switch5 : Switch  Criteria=u2 > Threshold  Threshold=false
  Switch6 : Switch  Criteria=u2 ~= 0
  Switch7 : Switch  Criteria=u2 > Threshold
  Switch8 : Switch  Criteria=u2 > Threshold
  Switch9 : Switch  Criteria=u2 > Threshold
  Triangle shift : Subsystem
  Triangle shift1 : Subsystem
  Triangle shift2 : Subsystem
  S1 : Outport  VectorParamsAs1DForOutWhenUnconnected=off
  S2 : Outport  Port=2  VectorParamsAs1DForOutWhenUnconnected=off
  S3 : Outport  Port=3  VectorParamsAs1DForOutWhenUnconnected=off
  S4 : Outport  Port=4  VectorParamsAs1DForOutWhenUnconnected=off
  S5 : Outport  Port=5  VectorParamsAs1DForOutWhenUnconnected=off
  S6 : Outport  Port=6  VectorParamsAs1DForOutWhenUnconnected=off
  PWM_en_rd_AXI : Outport  Port=7  VectorParamsAs1DForOutWhenUnconnected=off
  f_carrier_kHz_rd_AXI : Outport  Port=8  VectorParamsAs1DForOutWhenUnconnected=off
  T_carrier_us_rd_AXI : Outport  Port=9  VectorParamsAs1DForOutWhenUnconnected=off
  min_pulse_width_rd_AXI : Outport  Port=10  VectorParamsAs1DForOutWhenUnconnected=off
  enb_out : Outport  Port=11  VectorParamsAs1DForOutWhenUnconnected=off
  Triangle_Max : Outport  Port=12  VectorParamsAs1DForOutWhenUnconnected=off
  Triangle_Min : Outport  Port=13  VectorParamsAs1DForOutWhenUnconnected=off
  triangle_out : Outport  Port=14  VectorParamsAs1DForOutWhenUnconnected=off
  dir_out : Outport  Port=15  VectorParamsAs1DForOutWhenUnconnected=off
  wires:
  Constant7/1 -> Switch9/3
  Demux2/2 -> S6/1
  Constant8/1 -> Switch9/1
  Relational Operator2/1 -> Switch9/2
  Switch9/1 -> Switch5/1
  Demux/2 -> S2/1
  Relational Operator/1 -> Switch7/2
  Demux1/2 -> S4/1
  Constant5/1 -> Switch8/1
  Relational Operator1/1 -> Switch8/2
  Constant4/1 -> Switch8/3
  Constant1/1 -> Switch7/3
  Constant2/1 -> Switch7/1
  LimitPulseWidth/1(ref_sig_limit) -> Scope/2, Relational Operator/2
  LimitPulseWidth1/1(ref_sig_limit) -> Scope2/2, Relational Operator1/2
  LimitPulseWidth2/1(ref_sig_limit) -> Scope4/2, Relational Operator2/2
  Counter Ctrl/2(triangle_sig) -> triangle_out/1, Scope/1, Switch10/3
  PWM_en_AXI/1 -> Switch3/2, Switch5/2, Switch4/2, HDL Counter2/2, PWM_en_rd_AXI/1
  Delay/1 -> Switch/3
  Delay1/1 -> Switch1/3
  Delay2/1 -> Switch2/3
  Switch5/1 -> Demux2/1
  Switch8/1 -> Switch4/1
  Switch4/1 -> Demux1/1
  Switch3/1 -> Demux/1
  Constant10/1 -> Switch5/3, Switch3/3, Switch4/3
  U1_norm/1 -> Switch/1
  U3_norm/1 -> Switch2/1
  U2_norm/1 -> Switch1/1
  Counter Ctrl/1(dir_ctrl) -> dir_out/1, HDL Counter2/3, Scope10/1
  f_carrier_kHz_AXI/1 -> f_carrier_kHz_rd_AXI/1, Counter Ctrl/2(f_carrier_kHz)
  Relay1/1 -> Data Type Conversion1/1
  Data Type Conversion1/1 -> HDL Counter1/3
  HDL Counter1/1 -> Relay1/1
  Switch/1 -> Delay/1, LimitPulseWidth/1(ref_sig)
  Switch1/1 -> LimitPulseWidth1/1(ref_sig), Delay1/1
  Switch2/1 -> LimitPulseWidth2/1(ref_sig), Delay2/1
  Demux/1 -> Scope/3, S1/1
  Switch6/1 -> enb_out/1
  Constant11/1 -> Switch6/1
  Constant/1 -> Switch6/3
  Demux1/1 -> Scope2/3, S3/1
  Demux2/1 -> Scope4/3, S5/1
  T_carrier_us_AXI/1 -> T_carrier_us_rd_AXI/1, Counter Ctrl/3(T_carrier_us)
  Switch7/1 -> Switch3/1
  min_pulse_width_AXI/1 -> LimitPulseWidth/2(min_pulse_width), LimitPulseWidth2/2(min_pulse_width), LimitPulseWidth1/2(min_pulse_width), min_pulse_width_rd_AXI/1
  Counter Ctrl/3(Period_CenterMax) -> MinOrMax/1, Triangle_Max/1, Scope/4
  Counter Ctrl/4(Period_CenterMin) -> MinOrMax/2, Scope/5, Triangle_Min/1
  MinOrMax/1 -> Switch1/2, Switch2/2, Switch/2  "Allow (assymetrical) anew reference value"
  triangle_in/1 -> Delay4/1
  count_src_ext_AXI/1 -> Switch10/2
  HDL Counter2/1 -> Counter Ctrl/1(hdl_cnt)
  Delay4/1 -> Switch10/1
  triangle_shift_HB1_AXI/1 -> Triangle shift/2(triangle_shift)
  Triangle shift/1(triangle_sig) -> Relational Operator/1
  Triangle shift1/1(triangle_sig) -> Relational Operator1/1
  Switch10/1 -> Triangle shift/1(triangle_in), Triangle shift1/1(triangle_in), Triangle shift2/1(triangle_in), Scope4/1, Switch6/2, Scope2/1
  triangle_shift_HB2_AXI/1 -> Triangle shift1/2(triangle_shift)
  Triangle shift2/1(triangle_sig) -> Relational Operator2/1
  triangle_shift_HB3_AXI/1 -> Triangle shift2/2(triangle_shift)
  counter_reset/1 -> HDL Counter2/1

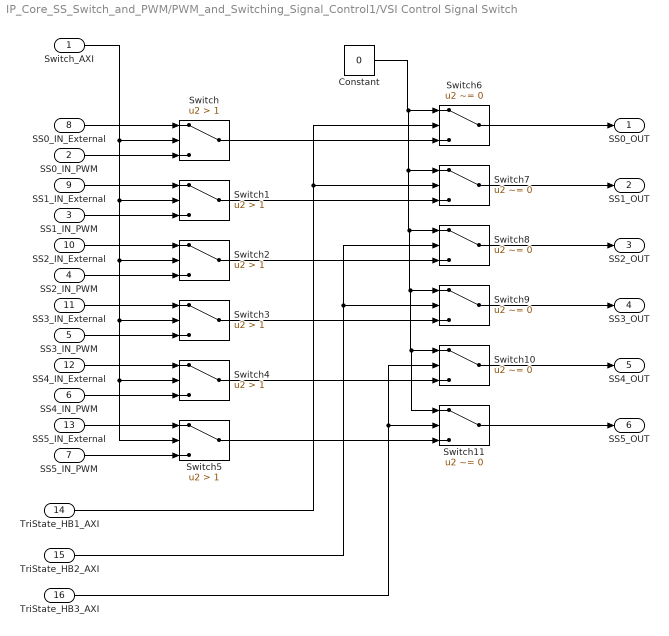
== system IP_Core_SS_Switch_and_PWM/PWM_and_Switching_Signal_Control1/VSI Control Signal Switch ==
  Switch_AXI : Inport
  SS0_IN_PWM : Inport  Port=2
  SS1_IN_PWM : Inport  Port=3
  SS2_IN_PWM : Inport  Port=4
  SS3_IN_PWM : Inport  Port=5
  SS4_IN_PWM : Inport  Port=6
  SS5_IN_PWM : Inport  Port=7
  SS0_IN_External : Inport  Port=8
  SS1_IN_External : Inport  Port=9
  SS2_IN_External : Inport  Port=10
  SS3_IN_External : Inport  Port=11
  SS4_IN_External : Inport  Port=12
  SS5_IN_External : Inport  Port=13
  TriState_HB1_AXI : Inport  Port=14
  TriState_HB2_AXI : Inport  Port=15
  TriState_HB3_AXI : Inport  Port=16
  Constant : Constant  Value=0  OutDataTypeStr=boolean  SampleTime=T_FPGA_clk
  Switch{,1..5} (6 alike) : Switch  Criteria=u2 > Threshold  Threshold=1
  Switch{6..11} (6 alike) : Switch  Criteria=u2 ~= 0  Threshold=1
  SS0_OUT : Outport  VectorParamsAs1DForOutWhenUnconnected=off
  SS1_OUT : Outport  Port=2  VectorParamsAs1DForOutWhenUnconnected=off
  SS2_OUT : Outport  Port=3  VectorParamsAs1DForOutWhenUnconnected=off
  SS3_OUT : Outport  Port=4  VectorParamsAs1DForOutWhenUnconnected=off
  SS4_OUT : Outport  Port=5  VectorParamsAs1DForOutWhenUnconnected=off
  SS5_OUT : Outport  Port=6  VectorParamsAs1DForOutWhenUnconnected=off
  wires:
  Switch_AXI/1 -> Switch4/2, Switch5/2, Switch3/2, Switch2/2, Switch1/2, Switch/2
  Switch5/1 -> Switch11/3
  Switch/1 -> Switch6/3
  Switch3/1 -> Switch9/3
  Switch2/1 -> Switch8/3
  Switch1/1 -> Switch7/3
  Switch4/1 -> Switch10/3
  SS0_IN_PWM/1 -> Switch/3
  SS0_IN_External/1 -> Switch/1
  SS1_IN_External/1 -> Switch1/1
  SS1_IN_PWM/1 -> Switch1/3
  SS2_IN_External/1 -> Switch2/1
  SS2_IN_PWM/1 -> Switch2/3
  SS3_IN_External/1 -> Switch3/1
  SS3_IN_PWM/1 -> Switch3/3
  SS4_IN_External/1 -> Switch4/1
  SS4_IN_PWM/1 -> Switch4/3
  SS5_IN_External/1 -> Switch5/1
  SS5_IN_PWM/1 -> Switch5/3
  TriState_HB3_AXI/1 -> Switch10/2, Switch11/2
  TriState_HB2_AXI/1 -> Switch8/2, Switch9/2
  TriState_HB1_AXI/1 -> Switch6/2, Switch7/2
  Switch11/1 -> SS5_OUT/1
  Switch10/1 -> SS4_OUT/1
  Switch9/1 -> SS3_OUT/1
  Switch8/1 -> SS2_OUT/1
  Switch7/1 -> SS1_OUT/1
  Switch6/1 -> SS0_OUT/1
  Constant/1 -> Switch11/1, Switch10/1, Switch9/1, Switch8/1, Switch7/1, Switch6/1

== system IP_Core_SS_Switch_and_PWM/PWM_and_Switching_Signal_Control/GenPWM/Counter Ctrl ==
  note: if (hdl_cnt >= step_cnt)
      | 	dir_ctrl = true;
      | else if (hdl_cnt <= 0)
      | 	dir_ctrl = false;
      | else
      | 	dir_ctrl = dir_ctrl;
  note: scaling triangle amplitude to 100
  hdl_cnt : Inport
  f_carrier_kHz : Inport  Port=2
  T_carrier_us : Inport  Port=3
  Constant1 : Constant  Value=0  OutDataTypeStr=fixdt(0,20,0)  SampleTime=T_FPGA_clk
  Constant11 : Constant  Value=0  OutDataTypeStr=fixdt(0,20,0)  SampleTime=T_FPGA_clk
  Constant12 : Constant  Value=false  SampleTime=T_FPGA_clk
  Constant14 : Constant  Value=true  SampleTime=T_FPGA_clk
  Delay : Delay  DelayLength=1
  Delay6 : Delay  DelayLength=1
  Logical Operator : Logic  Operator=OR  AllPortsSameDT=off  OutDataTypeStr=boolean
  Product : Product  OutDataTypeStr=fixdt(0,18,17)
  Relational Operator1 : RelationalOperator  Operator===  OutDataTypeStr=boolean  RndMeth=Nearest
  Relational Operator2 : RelationalOperator  Operator===  OutDataTypeStr=boolean  RndMeth=Nearest
  Relational Operator4 : RelationalOperator  OutDataTypeStr=boolean  RndMeth=Nearest
  Relational Operator5 : RelationalOperator  Operator=<=  OutDataTypeStr=boolean  RndMeth=Nearest
  Scope9 : Scope  NumInputPorts=2
  Switch6 : Switch  Criteria=u2 > Threshold
  Switch7 : Switch  Criteria=u2 > Threshold
  dir_ctrl : Outport  VectorParamsAs1DForOutWhenUnconnected=off
  triangle_sig : Outport  Port=2  VectorParamsAs1DForOutWhenUnconnected=off
  Period_CenterMax : Outport  Port=3  VectorParamsAs1DForOutWhenUnconnected=off
  Period_CenterMin : Outport  Port=4  VectorParamsAs1DForOutWhenUnconnected=off
  wires:
  hdl_cnt/1 -> Relational Operator2/1, Relational Operator1/1, Relational Operator5/1, Relational Operator4/1, Product/1, Scope9/1
  Switch6/1 -> Delay6/1, dir_ctrl/1
  Relational Operator4/1 -> Switch7/2, Logical Operator/1
  Relational Operator5/1 -> Logical Operator/2
  Constant11/1 -> Relational Operator5/2
  Logical Operator/1 -> Switch6/2
  Switch7/1 -> Switch6/1
  Constant12/1 -> Switch7/1
  Constant14/1 -> Switch7/3
  Delay6/1 -> Switch6/3
  T_carrier_us/1 -> Relational Operator4/2, Relational Operator1/2
  f_carrier_kHz/1 -> Delay/1
  Delay/1 -> Scope9/2, Product/2
  Relational Operator1/1 -> Period_CenterMax/1
  Relational Operator2/1 -> Period_CenterMin/1
  Constant1/1 -> Relational Operator2/2
  Product/1 -> triangle_sig/1

== system IP_Core_SS_Switch_and_PWM/PWM_and_Switching_Signal_Control/GenPWM/LimitPulseWidth ==
  note: Set pulse width between 0-1
  ref_sig : Inport
  min_pulse_width : Inport  Port=2
  Add : Sum  Inputs=+-  OutDataTypeStr=Inherit: Same as first input
  Constant : Constant  OutDataTypeStr=fixdt(1,18,16)  SampleTime=T_FPGA_clk
  Constant1 : Constant  Value=1.01  OutDataTypeStr=fixdt(1,18,16)  SampleTime=T_FPGA_clk
  Constant2 : Constant  Value=0  OutDataTypeStr=fixdt(1,18,16)  SampleTime=T_FPGA_clk
  Logical Operator : Logic  Operator=OR  AllPortsSameDT=off  OutDataTypeStr=boolean
  Relational Operator : RelationalOperator  Operator=>  OutDataTypeStr=boolean  RndMeth=Nearest
  Relational Operator1 : RelationalOperator  Operator=<  OutDataTypeStr=boolean  RndMeth=Nearest
  Saturation : Saturate  UpperLimit=1  LowerLimit=0  OutDataTypeStr=fixdt(1,18,16)
  Switch1 : Switch  Criteria=u2 > Threshold
  Switch6 : Switch  Criteria=u2 > Threshold
  ref_sig_limit : Outport  VectorParamsAs1DForOutWhenUnconnected=off
  wires:
  Constant/1 -> Add/1
  min_pulse_width/1 -> Add/2, Saturation/1
  Add/1 -> Relational Operator/2
  ref_sig/1 -> Switch6/3, Relational Operator/1, Relational Operator1/1
  Relational Operator/1 -> Logical Operator/1
  Relational Operator1/1 -> Logical Operator/2, Switch1/2
  Logical Operator/1 -> Switch6/2
  Constant1/1 -> Switch1/3
  Switch1/1 -> Switch6/1
  Constant2/1 -> Switch1/1
  Switch6/1 -> ref_sig_limit/1
  Saturation/1 -> Relational Operator1/2

== system IP_Core_SS_Switch_and_PWM/PWM_and_Switching_Signal_Control/GenPWM/LimitPulseWidth1 ==
  note: Set pulse width in percent
  ref_sig : Inport
  min_pulse_width : Inport  Port=2
  Add : Sum  Inputs=+-  OutDataTypeStr=Inherit: Same as first input
  Constant : Constant  OutDataTypeStr=fixdt(1,18,16)  SampleTime=T_FPGA_clk
  Constant1 : Constant  Value=1.01  OutDataTypeStr=fixdt(1,18,16)  SampleTime=T_FPGA_clk
  Constant2 : Constant  Value=0  OutDataTypeStr=fixdt(1,18,16)  SampleTime=T_FPGA_clk
  Logical Operator : Logic  Operator=OR  AllPortsSameDT=off  OutDataTypeStr=boolean
  Relational Operator : RelationalOperator  Operator=>  OutDataTypeStr=boolean  RndMeth=Nearest
  Relational Operator1 : RelationalOperator  Operator=<  OutDataTypeStr=boolean  RndMeth=Nearest
  Saturation : Saturate  UpperLimit=1  LowerLimit=0  OutDataTypeStr=fixdt(1,18,16)
  Switch1 : Switch  Criteria=u2 > Threshold
  Switch6 : Switch  Criteria=u2 > Threshold
  ref_sig_limit : Outport  VectorParamsAs1DForOutWhenUnconnected=off
  wires:
  Constant/1 -> Add/1
  min_pulse_width/1 -> Add/2, Saturation/1
  Add/1 -> Relational Operator/2
  ref_sig/1 -> Switch6/3, Relational Operator/1, Relational Operator1/1
  Relational Operator/1 -> Logical Operator/1
  Relational Operator1/1 -> Logical Operator/2, Switch1/2
  Logical Operator/1 -> Switch6/2
  Constant1/1 -> Switch1/3
  Switch1/1 -> Switch6/1
  Constant2/1 -> Switch1/1
  Switch6/1 -> ref_sig_limit/1
  Saturation/1 -> Relational Operator1/2
